simulink model "comparando_bloco_FCEM"  (R2012b)
settings: Solver=ode45  StartTime=0.0  StopTime=3  RelTol=1e-3
undefined symbols (not defined in the file): Ke, KE
libraries: simulink x2
settings Model: Creator=Juliano  LastModifiedBy=Juliano

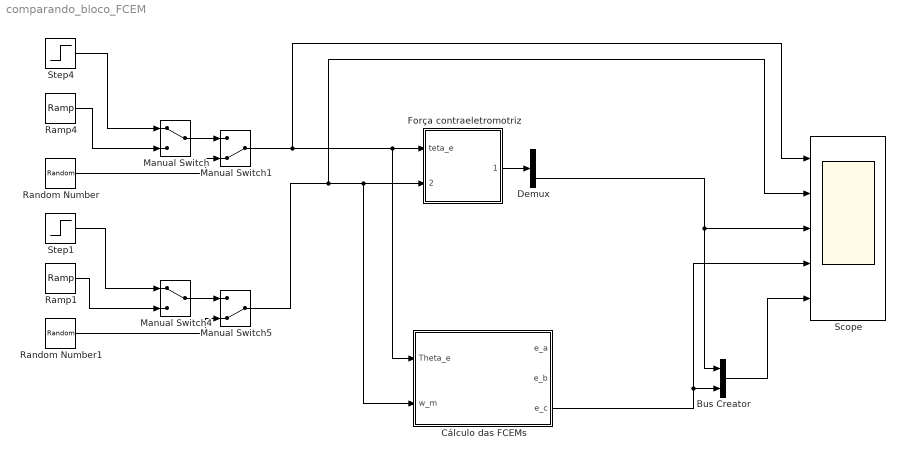
== system comparando_bloco_FCEM ==
  Bus Creator : BusCreator  Inputs=2
  Cálculo das FCEMs : Subsystem
  Demux : Demux  Outputs=3
  Força contraeletromotriz : Subsystem
  Manual Switch : ManualSwitch
  Manual Switch1 : ManualSwitch  CurrentSetting=0
  Manual Switch4 : ManualSwitch
  Manual Switch5 : ManualSwitch  CurrentSetting=0
  Ramp1 : simulink/Sources/Ramp  slope=20  start=0  X0=0
  Ramp4 : simulink/Sources/Ramp  slope=2*pi  start=0  X0=0
  Random Number : RandomNumber  Variance=20  SampleTime=0.1
  Random Number1 : RandomNumber  Variance=20  Seed=1  SampleTime=0.1
  Scope : Scope  NumInputPorts=5
      settings: TimeRange=0.5  YMin=0~0~0~-5~-5  YMax=800000~800000~800000~5~5
  Step1 : Step  Time=0  After=20  SampleTime=0
  Step4 : Step  Time=0  After=-3.115  SampleTime=0
  wires:
  Manual Switch/1 -> Manual Switch1/1
  Manual Switch4/1 -> Manual Switch5/1
  Step4/1 -> Manual Switch/1
  Ramp4/1 -> Manual Switch/2
  Random Number/1 -> Manual Switch1/2
  Manual Switch5/1 -> Scope/2, Cálculo das FCEMs/2(w_m), Força contraeletromotriz/2(omega_e)
  Bus Creator/1 -> Scope/5
  Manual Switch1/1 -> Scope/1, Cálculo das FCEMs/1(Theta_e), Força contraeletromotriz/1(teta_e)
  Step1/1 -> Manual Switch4/1
  Ramp1/1 -> Manual Switch4/2
  Random Number1/1 -> Manual Switch5/2
  Demux/3 -> Scope/3, Bus Creator/1
  Cálculo das FCEMs/3(e_c) -> Scope/4, Bus Creator/2
  Força contraeletromotriz/1(Fcem abc) -> Demux/1

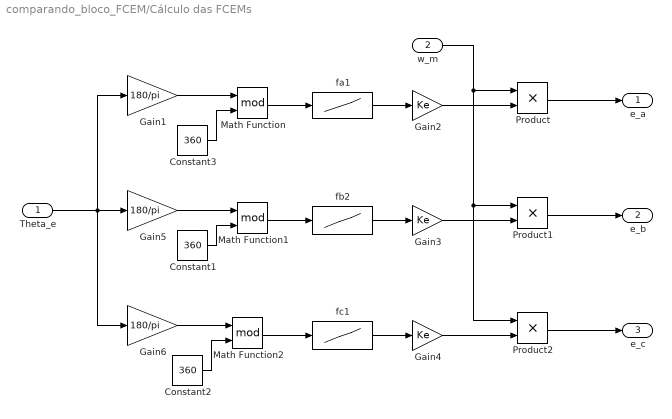
== system comparando_bloco_FCEM/Cálculo das FCEMs ==
  Theta_e : Inport
  w_m : Inport  Port=2
  Constant1 : Constant  Value=360
  Constant2 : Constant  Value=360
  Constant3 : Constant  Value=360
  Gain1 : Gain  Gain=180/pi
  Gain2 : Gain  Gain=Ke
  Gain3 : Gain  Gain=Ke
  Gain4 : Gain  Gain=Ke
  Gain5 : Gain  Gain=180/pi
  Gain6 : Gain  Gain=180/pi
  Math Function : Math  Operator=mod  SaturateOnIntegerOverflow=on
  Math Function1 : Math  Operator=mod  SaturateOnIntegerOverflow=on
  Math Function2 : Math  Operator=mod  SaturateOnIntegerOverflow=on
  Product : Product  RndMeth=Zero
  Product1 : Product  RndMeth=Zero
  Product2 : Product  RndMeth=Zero
  fa1 : Lookup  InputValues=[0 30 60 90 120 150 180 210 240 270 300 330 360]  Table=[ 1 1 1 0 -1 -1 -1 -1 -1 0 1 1 1]
  fb2 : Lookup  InputValues=[0 30 60 90 120 150 180 210 240 270 300 330 360]  Table=[-1 0 1 1 1 1 1 0 -1 -1 -1 -1 -1]
  fc1 : Lookup  InputValues=[0 30 60 90 120 150 180 210 240 270 300 330 360]  Table=[-1 -1 -1 -1 -1 0 1 1 1 1 1 0 -1]
  e_a : Outport
  e_b : Outport  Port=2
  e_c : Outport  Port=3
  wires:
  fc1/1 -> Gain4/1
  Math Function2/1 -> fc1/1
  fb2/1 -> Gain3/1
  Math Function1/1 -> fb2/1
  fa1/1 -> Gain2/1
  Math Function/1 -> fa1/1
  Gain6/1 -> Math Function2/1
  Gain5/1 -> Math Function1/1
  Gain1/1 -> Math Function/1
  Gain4/1 -> Product2/2
  Gain3/1 -> Product1/2
  w_m/1 -> Product2/1, Product1/1, Product/1
  Gain2/1 -> Product/2
  Product2/1 -> e_c/1
  Theta_e/1 -> Gain6/1, Gain1/1, Gain5/1
  Product1/1 -> e_b/1
  Product/1 -> e_a/1
  Constant3/1 -> Math Function/2
  Constant1/1 -> Math Function1/2
  Constant2/1 -> Math Function2/2

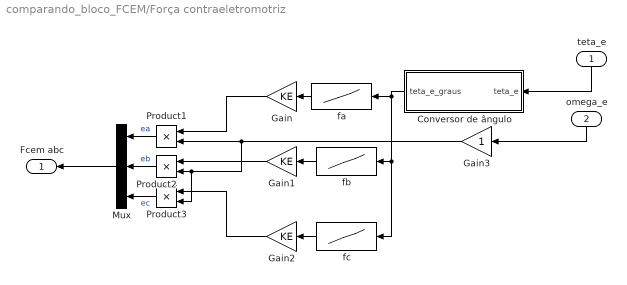
== system comparando_bloco_FCEM/Força contraeletromotriz ==
  teta_e : Inport
  omega_e : Inport  Port=2
  Conversor de ângulo : Subsystem
  Gain : Gain  Gain=KE
  Gain1 : Gain  Gain=KE
  Gain2 : Gain  Gain=KE
  Gain3 : Gain
  Mux : Mux  Inputs=3
  Product1 : Product  SaturateOnIntegerOverflow=on  OutDataTypeStr=Inherit: Same as first input
  Product2 : Product  SaturateOnIntegerOverflow=on  OutDataTypeStr=Inherit: Same as first input
  Product3 : Product  SaturateOnIntegerOverflow=on  OutDataTypeStr=Inherit: Same as first input
  fa : Lookup  InputValues=[-180 -150 -120 -90 -60 -30 0 30 60 90 120 150 180]  Table=[-1 -1 -1 0 1 1 1 1 1 0 -1 -1 -1]
  fb : Lookup  InputValues=[-180 -150 -120 -90 -60 -30 0 30 60 90 120 150 180]  Table="[1 0 -1 -1 -1 -1  -1 0 1 1 1 1 1]"
  fc : Lookup  InputValues=[-180 -150 -120 -90 -60 -30 0 30 60 90 120 150 180]  Table=[1 1 1 1 1 0 -1 -1 -1 -1 -1 0 1]
  Fcem abc : Outport
  wires:
  Gain3/1 -> Product3/2, Product2/2, Product1/2
  omega_e/1 -> Gain3/1
  Gain2/1 -> Product3/1
  Gain1/1 -> Product2/1
  Gain/1 -> Product1/1
  Product3/1 -> Mux/3  "ec"
  Product2/1 -> Mux/2  "eb"
  Product1/1 -> Mux/1  "ea"
  Conversor de ângulo/1(teta_e_graus) -> fb/1, fc/1, fa/1
  Mux/1 -> Fcem abc/1
  teta_e/1 -> Conversor de ângulo/1(teta_e)
  fc/1 -> Gain2/1
  fb/1 -> Gain1/1
  fa/1 -> Gain/1

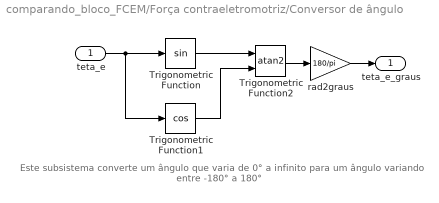
== system comparando_bloco_FCEM/Força contraeletromotriz/Conversor de ângulo ==
  note: Este subsistema converte um ângulo que varia de 0° a infinito
      | para um ângulo variando entre -180° a 180°
  teta_e : Inport
  Trigonometric Function : Trigonometry
  Trigonometric Function1 : Trigonometry  Operator=cos
  Trigonometric Function2 : Trigonometry  Operator=atan2
  rad2graus : Gain  Gain=180/pi  SaturateOnIntegerOverflow=on  OutDataTypeStr=Inherit: Same as input  ParamDataTypeStr=Inherit: Same as input
  teta_e_graus : Outport
  wires:
  rad2graus/1 -> teta_e_graus/1
  Trigonometric Function2/1 -> rad2graus/1
  Trigonometric Function1/1 -> Trigonometric Function2/2
  Trigonometric Function/1 -> Trigonometric Function2/1
  teta_e/1 -> Trigonometric Function1/1, Trigonometric Function/1
